simulink model "DSimulator_robot1DOFV_NG"  (R2021a)
settings: Solver=ode1  StartTime=0.0  StopTime=500  FixedStep=0.004  RelTol=1e-3  EnableMultiTasking=on
undefined symbols (not defined in the file or in its folder): Dinamic_robot1DOFV, Tau
settings Model: Creator=E. Dean  LastModifiedBy=dean
settings SolverCC: AlgebraicLoopSolver=TrustRegion
settings DataIOCC: LimitDataPoints=on  SaveFormat=Array  SignalLoggingSaveFormat=ModelDataLogs  ReturnWorkspaceOutputs=off
settings OptimizationCC: ExpressionDepthLimit=2147483647  LifeSpan=inf
settings DebuggingCC: UnderspecifiedInitializationDetection=Classic  MergeDetectMultiDrivingBlocksExec=none  SolverPrmCheckMsg=warning  FcnCallInpInsideContextMsg=warning  StateNameClashWarn=warning  SFUnexpectedBacktrackingDiag=warning  SFNoUnconditionalDefaultTransitionDiag=warning  SFExecutionAtInitializationDiag=none  SFMachineParentedDataDiag=warning  ArithmeticOperatorsInVariantConditions=warning
settings HardwareCC: ProdBitPerPointer=32  ProdBitPerSizeT=32  ProdBitPerPtrDiffT=32  ProdLargestAtomicFloat=None  ProdIntDivRoundTo=Undefined  ProdEndianess=Unspecified  ProdWordSize=32  ProdHWDeviceType=32-bit Generic
settings ModelReferenceCC: PropagateSignalLabelsOutOfModel=off
settings SFSimCC: SimUseLocalCustomCode=off  CustomCodeUndefinedFunction=UseInterfaceOnly
settings RTWCC: RTWUseLocalCustomCode=off
settings CodeAppCC: StateflowObjectComments=on
settings GRTTargetCC: TargetLangStandard=C89/C90 (ANSI)  CombineOutputUpdateFcns=off  GRTInterface=on
settings ConfigComp: CovMetricSettings=dw  CovSaveCumulativeToWorkspaceVar=on  CovSaveSingleToWorkspaceVar=on

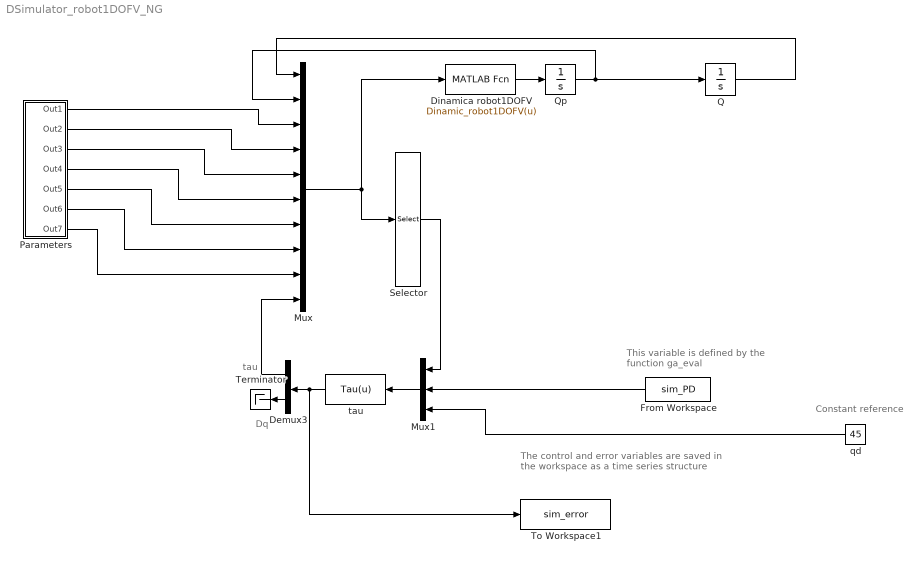
== system DSimulator_robot1DOFV_NG ==
  note: Constant reference
  note: tau
  note: Dq
  note: The control and error variables are saved
      | in the workspace as
      | a time series structure
  note: This variable is defined
      | by the function ga_eval
  Demux3 : Demux  Outputs=2
  Dinamica robot1DOFV : MATLABFcn  MATLABFcn=Dinamic_robot1DOFV(u)  OutputDimensions=1
  From Workspace : FromWorkspace  VariableName=sim_PD
  Mux : Mux  Inputs=10
  Mux1 : Mux  Inputs=3
  Parameters : Subsystem
  Q : Integrator
  Qp : Integrator  InitialCondition=[0]
  Selector : Selector  InputPortWidth=13  IndexOptions=Index vector (dialog)  Indices=[1:12]  OutputSizes=1
  Terminator : Terminator
  To Workspace1 : ToWorkspace  VariableName=sim_error  SaveFormat=Timeseries  SampleTime=-1
  qd : Constant  Value=45
  tau : MATLABFcn  MATLABFcn=Tau(u)  OutputDimensions=2
  wires:
  Qp/1 -> Q/1, Mux/2
  Mux/1 -> Selector/1, Dinamica robot1DOFV/1
  Mux1/1 -> tau/1
  Selector/1 -> Mux1/1
  qd/1 -> Mux1/3
  Dinamica robot1DOFV/1 -> Qp/1
  tau/1 -> To Workspace1/1, Demux3/1
  Demux3/1 -> Mux/10
  Demux3/2 -> Terminator/1
  Q/1 -> Mux/1
  From Workspace/1 -> Mux1/2
  Parameters/1(Out1) -> Mux/3
  Parameters/2(Out2) -> Mux/4
  Parameters/3(Out3) -> Mux/5
  Parameters/4(Out4) -> Mux/6
  Parameters/5(Out5) -> Mux/7
  Parameters/6(Out6) -> Mux/8
  Parameters/7(Out7) -> Mux/9

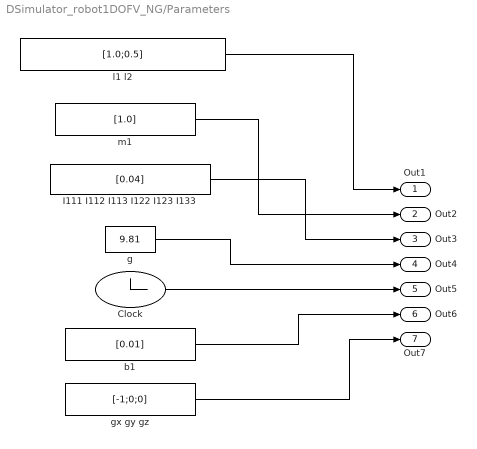
== system DSimulator_robot1DOFV_NG/Parameters ==
  Clock : Clock
  I111 I112 I113 I122 I123 I133 : Constant  Value=[0.04]
  "b1 " : Constant  Value=[0.01]
  g : Constant  Value=9.81
  gx gy gz : Constant  Value=[-1;0;0]
  "l1 l2 " : Constant  Value=[1.0;0.5]
  "m1 " : Constant  Value=[1.0]
  Out1 : Outport
  Out2 : Outport  Port=2
  Out3 : Outport  Port=3
  Out4 : Outport  Port=4
  Out5 : Outport  Port=5
  Out6 : Outport  Port=6
  Out7 : Outport  Port=7
  wires:
  gx gy gz/1 -> Out7/1
  I111 I112 I113 I122 I123 I133/1 -> Out3/1
  "m1 "/1 -> Out2/1
  "l1 l2 "/1 -> Out1/1
  "b1 "/1 -> Out6/1
  Clock/1 -> Out5/1
  g/1 -> Out4/1
